simulink model "quadplane_sim"  (R2023a)
settings: Solver=FixedStepAuto  StartTime=0.0  StopTime=5  FixedStep=0.00001  RelTol=1e-6
values from neighbouring files (symbols this model uses):
  framePeriod_s = 1/frameRate_hz    (= 0.02)    [setup.m]
undefined symbols (not defined in the file or in its folder): Aircraft, datetime, datevec, Earth, Env, Fmu, InitCond, Telem, WGS84
libraries: simulink x9, aerolibconvert2 x5, aerolibasang x3, aerolibtransform2 x2, aerolibatmos2 x1, aerolibgravity2 x1, sharedtransform x1, uavutilslib x1, aerolibadyn x1, shared6dof x1
(part 4 of 4)

== system quadplane_sim/Flight Management Unit/Control Laws/Variant Subsystem/FMU v2/Virtual to Non-Virtual Mapping4/Subsystem2 ==
  Non-Virtual : Inport  OutDataTypeStr=Bus: AnalogData
  Bus Creator : BusCreator  Inputs=1
  Bus Selector : BusSelector  OutputSignals=val
  Data Type Conversion : DataTypeConversion  OutDataTypeStr=double  SaturateOnIntegerOverflow=off  RndMeth=Floor
  Virtual : Outport
  wires:
  Non-Virtual/1 -> Bus Selector/1
  Bus Creator/1 -> Virtual/1
  Data Type Conversion/1 -> Bus Creator/1  "Values"
  Bus Selector/1 -> Data Type Conversion/1  "<val>"

== system quadplane_sim/Flight Management Unit/Control Laws/Variant Subsystem/FMU v2/Virtual to Non-Virtual Mapping4/Subsystem3 ==
  Non-Virtual : Inport  OutDataTypeStr=Bus: PwmCmd
  Bus Creator : BusCreator  Inputs=2
  Bus Selector : BusSelector  OutputSignals=cnt,cmd
  Data Type Conversion : DataTypeConversion  OutDataTypeStr=double  SaturateOnIntegerOverflow=off  RndMeth=Floor
  Data Type Conversion1 : DataTypeConversion  OutDataTypeStr=double  SaturateOnIntegerOverflow=off  RndMeth=Floor
  Virtual : Outport
  wires:
  Non-Virtual/1 -> Bus Selector/1
  Bus Selector/2 -> Data Type Conversion1/1  "<cmd>"
  Data Type Conversion1/1 -> Bus Creator/2  "Cmds"
  Data Type Conversion/1 -> Bus Creator/1  "Cnt"
  Bus Selector/1 -> Data Type Conversion/1  "<cnt>"
  Bus Creator/1 -> Virtual/1

== system quadplane_sim/Flight Management Unit/Control Laws/Variant Subsystem/FMU v2/Virtual to Non-Virtual Mapping4/Subsystem4 ==
  Non-Virtual : Inport  OutDataTypeStr=Bus: SbusCmd
  Bus Creator : BusCreator  Inputs=4
  Bus Selector : BusSelector  OutputSignals=ch17,ch18,cnt,cmd
  Data Type Conversion{,1..3} (4 alike) : DataTypeConversion  OutDataTypeStr=double  SaturateOnIntegerOverflow=off  RndMeth=Floor
  Virtual : Outport
  wires:
  Non-Virtual/1 -> Bus Selector/1
  Bus Creator/1 -> Virtual/1
  Bus Selector/1 -> Data Type Conversion/1  "<ch17>"
  Bus Selector/2 -> Data Type Conversion1/1  "<ch18>"
  Bus Selector/3 -> Data Type Conversion2/1  "<cnt>"
  Bus Selector/4 -> Data Type Conversion3/1  "<cmd>"
  Data Type Conversion2/1 -> Bus Creator/3  "Cnt"
  Data Type Conversion3/1 -> Bus Creator/4  "Cmds"
  Data Type Conversion1/1 -> Bus Creator/2  "Ch 18"
  Data Type Conversion/1 -> Bus Creator/1  "Ch 17"

== system quadplane_sim/Flight Management Unit/Control Laws/Variant Subsystem/FMU v2/Virtual to Non-Virtual Mapping5/Virtual to Non-Virtual Mapping1 ==
  Virtual : Inport
  Bus Creator : BusCreator  Inputs=6
  Bus Selector : BusSelector  OutputSignals=New Data,Lost Frame,Failsafe,Ch 17,Ch 18,Channel Data
  Data Type Conversion{,1..4} (5 alike) : DataTypeConversion  OutDataTypeStr=boolean  SaturateOnIntegerOverflow=off  RndMeth=Floor
  Data Type Conversion5 : DataTypeConversion  OutDataTypeStr=int16  SaturateOnIntegerOverflow=off  RndMeth=Floor
  Non-Virtual : Outport  OutDataTypeStr=Bus: InceptorData
  wires:
  Virtual/1 -> Bus Selector/1
  Bus Creator/1 -> Non-Virtual/1
  Bus Selector/1 -> Data Type Conversion/1  "<New Data>"
  Bus Selector/2 -> Data Type Conversion1/1  "<Lost Frame>"
  Bus Selector/3 -> Data Type Conversion2/1  "<Failsafe>"
  Bus Selector/4 -> Data Type Conversion3/1  "<Ch 17>"
  Bus Selector/5 -> Data Type Conversion4/1  "<Ch 18>"
  Bus Selector/6 -> Data Type Conversion5/1  "<Channel Data>"
  Data Type Conversion/1 -> Bus Creator/1  "new_data"
  Data Type Conversion1/1 -> Bus Creator/2  "lost_frame"
  Data Type Conversion2/1 -> Bus Creator/3  "failsafe"
  Data Type Conversion3/1 -> Bus Creator/4  "ch17"
  Data Type Conversion4/1 -> Bus Creator/5  "ch18"
  Data Type Conversion5/1 -> Bus Creator/6  "ch"

== system quadplane_sim/Flight Management Unit/Control Laws/Variant Subsystem/FMU v2/Virtual to Non-Virtual Mapping5/Virtual to Non-Virtual Mapping2 ==
  Virtual : Inport
  Bus Creator : BusCreator  Inputs=8
  Bus Selector : BusSelector  OutputSignals=New IMU Data,New Magnetometer Data,IMU Healthy,Magnetometer Healthy,Die Temperature [C],Accelerometer [m/s/s],Gyro [rad/s],Magnetometer [uT]
  Data Type Conversion{,1..3} (4 alike) : DataTypeConversion  OutDataTypeStr=boolean  SaturateOnIntegerOverflow=off  RndMeth=Floor
  Data Type Conversion{4..7} (4 alike) : DataTypeConversion  OutDataTypeStr=single  SaturateOnIntegerOverflow=off  RndMeth=Floor
  Non-Virtual : Outport  OutDataTypeStr=Bus: ImuData
  wires:
  Bus Creator/1 -> Non-Virtual/1
  Virtual/1 -> Bus Selector/1
  Bus Selector/1 -> Data Type Conversion/1  "<New IMU Data>"
  Data Type Conversion/1 -> Bus Creator/1  "new_imu_data"
  Bus Selector/2 -> Data Type Conversion1/1  "<New Magnetometer Data>"
  Data Type Conversion1/1 -> Bus Creator/2  "new_mag_data"
  Bus Selector/3 -> Data Type Conversion2/1  "<IMU Healthy>"
  Data Type Conversion2/1 -> Bus Creator/3  "imu_healthy"
  Bus Selector/4 -> Data Type Conversion3/1  "<Magnetometer Healthy>"
  Data Type Conversion3/1 -> Bus Creator/4  "mag_healthy"
  Bus Selector/5 -> Data Type Conversion4/1  "<Die Temperature [C]>"
  Data Type Conversion4/1 -> Bus Creator/5  "die_temp_c"
  Bus Selector/6 -> Data Type Conversion5/1  "<Accelerometer [m/s/s]>"
  Bus Selector/7 -> Data Type Conversion6/1  "<Gyro [rad/s]>"
  Bus Selector/8 -> Data Type Conversion7/1  "<Magnetometer [uT]>"
  Data Type Conversion5/1 -> Bus Creator/6  "accel_mps2"
  Data Type Conversion6/1 -> Bus Creator/7  "gyro_radps"
  Data Type Conversion7/1 -> Bus Creator/8  "mag_ut"

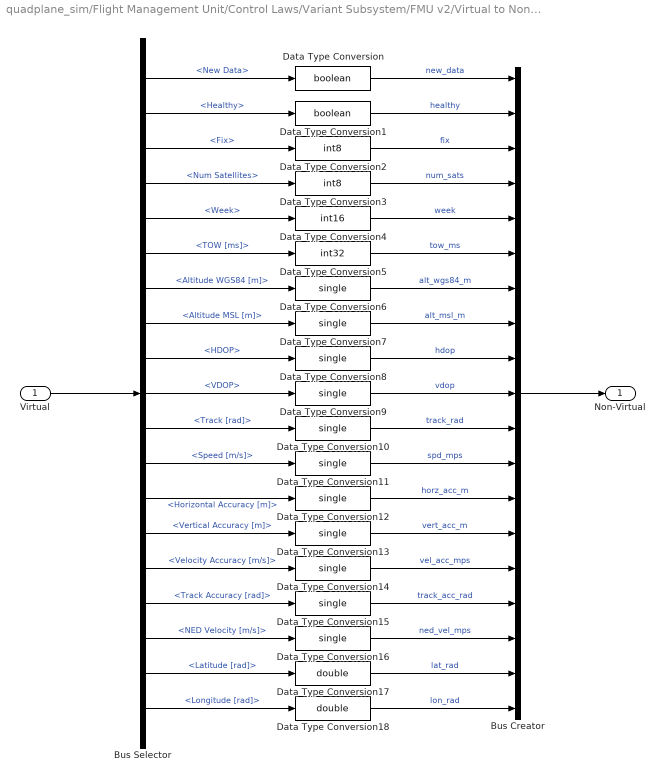
== system quadplane_sim/Flight Management Unit/Control Laws/Variant Subsystem/FMU v2/Virtual to Non-Virtual Mapping5/Virtual to Non-Virtual Mapping3 ==
  Virtual : Inport
  Bus Creator : BusCreator  Inputs=19
  Bus Selector : BusSelector  OutputSignals=New Data,Healthy,Fix,Num Satellites,Week,TOW [ms],Altitude WGS84 [m],Altitude MSL [m],HDOP,VDOP,Track [rad],Speed [m/s],Horizontal Accuracy [m],Vertical Accuracy [m],Velocity Accuracy [m/s],Track Accuracy [rad],NED Velocity [m/s],Latitude [rad],Longitude [rad]
  Data Type Conversion : DataTypeConversion  OutDataTypeStr=boolean  SaturateOnIntegerOverflow=off  RndMeth=Floor
  Data Type Conversion1 : DataTypeConversion  OutDataTypeStr=boolean  SaturateOnIntegerOverflow=off  RndMeth=Floor
  Data Type Conversion{6..16} (11 alike) : DataTypeConversion  OutDataTypeStr=single  SaturateOnIntegerOverflow=off  RndMeth=Floor
  Data Type Conversion17 : DataTypeConversion  OutDataTypeStr=double  SaturateOnIntegerOverflow=off  RndMeth=Floor
  Data Type Conversion18 : DataTypeConversion  OutDataTypeStr=double  SaturateOnIntegerOverflow=off  RndMeth=Floor
  Data Type Conversion2 : DataTypeConversion  OutDataTypeStr=int8  SaturateOnIntegerOverflow=off  RndMeth=Floor
  Data Type Conversion3 : DataTypeConversion  OutDataTypeStr=int8  SaturateOnIntegerOverflow=off  RndMeth=Floor
  Data Type Conversion4 : DataTypeConversion  OutDataTypeStr=int16  SaturateOnIntegerOverflow=off  RndMeth=Floor
  Data Type Conversion5 : DataTypeConversion  OutDataTypeStr=int32  SaturateOnIntegerOverflow=off  RndMeth=Floor
  Non-Virtual : Outport  OutDataTypeStr=Bus: GnssData
  wires:
  Virtual/1 -> Bus Selector/1
  Bus Creator/1 -> Non-Virtual/1
  Bus Selector/1 -> Data Type Conversion/1  "<New Data>"
  Data Type Conversion/1 -> Bus Creator/1  "new_data"
  Bus Selector/2 -> Data Type Conversion1/1  "<Healthy>"
  Data Type Conversion1/1 -> Bus Creator/2  "healthy"
  Bus Selector/3 -> Data Type Conversion2/1  "<Fix>"
  Data Type Conversion2/1 -> Bus Creator/3  "fix"
  Bus Selector/4 -> Data Type Conversion3/1  "<Num Satellites>"
  Data Type Conversion3/1 -> Bus Creator/4  "num_sats"
  Bus Selector/5 -> Data Type Conversion4/1  "<Week>"
  Data Type Conversion4/1 -> Bus Creator/5  "week"
  Bus Selector/6 -> Data Type Conversion5/1  "<TOW [ms]>"
  Data Type Conversion5/1 -> Bus Creator/6  "tow_ms"
  Bus Selector/7 -> Data Type Conversion6/1  "<Altitude WGS84 [m]>"
  Bus Selector/8 -> Data Type Conversion7/1  "<Altitude MSL [m]>"
  Data Type Conversion6/1 -> Bus Creator/7  "alt_wgs84_m"
  Data Type Conversion7/1 -> Bus Creator/8  "alt_msl_m"
  Bus Selector/9 -> Data Type Conversion8/1  "<HDOP>"
  Bus Selector/10 -> Data Type Conversion9/1  "<VDOP>"
  Data Type Conversion8/1 -> Bus Creator/9  "hdop"
  Data Type Conversion9/1 -> Bus Creator/10  "vdop"
  Bus Selector/11 -> Data Type Conversion10/1  "<Track [rad]>"
  Bus Selector/12 -> Data Type Conversion11/1  "<Speed [m/s]>"
  Data Type Conversion10/1 -> Bus Creator/11  "track_rad"
  Data Type Conversion11/1 -> Bus Creator/12  "spd_mps"
  Bus Selector/13 -> Data Type Conversion12/1  "<Horizontal Accuracy [m]>"
  Bus Selector/14 -> Data Type Conversion13/1  "<Vertical Accuracy [m]>"
  Bus Selector/15 -> Data Type Conversion14/1  "<Velocity Accuracy [m/s]>"
  Bus Selector/16 -> Data Type Conversion15/1  "<Track Accuracy [rad]>"
  Bus Selector/17 -> Data Type Conversion16/1  "<NED Velocity [m/s]>"
  Bus Selector/18 -> Data Type Conversion17/1  "<Latitude [rad]>"
  Bus Selector/19 -> Data Type Conversion18/1  "<Longitude [rad]>"
  Data Type Conversion18/1 -> Bus Creator/19  "lon_rad"
  Data Type Conversion17/1 -> Bus Creator/18  "lat_rad"
  Data Type Conversion16/1 -> Bus Creator/17  "ned_vel_mps"
  Data Type Conversion15/1 -> Bus Creator/16  "track_acc_rad"
  Data Type Conversion14/1 -> Bus Creator/15  "vel_acc_mps"
  Data Type Conversion13/1 -> Bus Creator/14  "vert_acc_m"
  Data Type Conversion12/1 -> Bus Creator/13  "horz_acc_m"

== system quadplane_sim/Flight Management Unit/Control Laws/Variant Subsystem/FMU v2/Virtual to Non-Virtual Mapping5/Virtual to Non-Virtual Mapping4 ==
  Virtual : Inport
  Bus Creator : BusCreator  Inputs=4
  Bus Selector : BusSelector  OutputSignals=New Data,Healthy,Pressure [Pa],Die Temperature [C]
  Data Type Conversion : DataTypeConversion  OutDataTypeStr=boolean  SaturateOnIntegerOverflow=off  RndMeth=Floor
  Data Type Conversion1 : DataTypeConversion  OutDataTypeStr=boolean  SaturateOnIntegerOverflow=off  RndMeth=Floor
  Data Type Conversion2 : DataTypeConversion  OutDataTypeStr=single  SaturateOnIntegerOverflow=off  RndMeth=Floor
  Data Type Conversion3 : DataTypeConversion  OutDataTypeStr=single  SaturateOnIntegerOverflow=off  RndMeth=Floor
  Non-Virtual : Outport  OutDataTypeStr=Bus: PresData
  wires:
  Bus Creator/1 -> Non-Virtual/1
  Virtual/1 -> Bus Selector/1
  Bus Selector/1 -> Data Type Conversion/1  "<New Data>"
  Data Type Conversion/1 -> Bus Creator/1  "new_data"
  Bus Selector/2 -> Data Type Conversion1/1  "<Healthy>"
  Data Type Conversion1/1 -> Bus Creator/2  "healthy"
  Bus Selector/3 -> Data Type Conversion2/1  "<Pressure [Pa]>"
  Data Type Conversion2/1 -> Bus Creator/3  "pres_pa"
  Bus Selector/4 -> Data Type Conversion3/1  "<Die Temperature [C]>"
  Data Type Conversion3/1 -> Bus Creator/4  "die_temp_c"

== system quadplane_sim/Flight Management Unit/Control Laws/Variant Subsystem/FMU v2/Virtual to Non-Virtual Mapping5/Virtual to Non-Virtual Mapping5 ==
  Virtual : Inport
  Bus Creator : BusCreator  Inputs=4
  Bus Selector : BusSelector  OutputSignals=New Data,Healthy,Pressure [Pa],Die Temperature [C]
  Data Type Conversion : DataTypeConversion  OutDataTypeStr=boolean  SaturateOnIntegerOverflow=off  RndMeth=Floor
  Data Type Conversion1 : DataTypeConversion  OutDataTypeStr=boolean  SaturateOnIntegerOverflow=off  RndMeth=Floor
  Data Type Conversion2 : DataTypeConversion  OutDataTypeStr=single  SaturateOnIntegerOverflow=off  RndMeth=Floor
  Data Type Conversion3 : DataTypeConversion  OutDataTypeStr=single  SaturateOnIntegerOverflow=off  RndMeth=Floor
  Non-Virtual : Outport  OutDataTypeStr=Bus: PresData
  wires:
  Data Type Conversion3/1 -> Bus Creator/4  "die_temp_c"
  Bus Selector/4 -> Data Type Conversion3/1  "<Die Temperature [C]>"
  Data Type Conversion2/1 -> Bus Creator/3  "pres_pa"
  Bus Selector/3 -> Data Type Conversion2/1  "<Pressure [Pa]>"
  Data Type Conversion1/1 -> Bus Creator/2  "healthy"
  Bus Selector/2 -> Data Type Conversion1/1  "<Healthy>"
  Data Type Conversion/1 -> Bus Creator/1  "new_data"
  Bus Selector/1 -> Data Type Conversion/1  "<New Data>"
  Virtual/1 -> Bus Selector/1
  Bus Creator/1 -> Non-Virtual/1

== system quadplane_sim/Flight Management Unit/Control Laws/Variant Subsystem/FMU v2/Virtual to Non-Virtual Mapping5/Virtual to Non-Virtual Mapping6 ==
  Virtual : Inport
  Bus Creator : BusCreator  Inputs=1
  Bus Selector : BusSelector  OutputSignals=Voltages
  Data Type Conversion2 : DataTypeConversion  OutDataTypeStr=single  SaturateOnIntegerOverflow=off  RndMeth=Floor
  Non-Virtual : Outport  OutDataTypeStr=Bus: AdcData
  wires:
  Bus Creator/1 -> Non-Virtual/1
  Virtual/1 -> Bus Selector/1
  Data Type Conversion2/1 -> Bus Creator/1  "volt"
  Bus Selector/1 -> Data Type Conversion2/1  "<Voltages>"

== system quadplane_sim/Flight Management Unit/Control Laws/Variant Subsystem/FMU v2/Virtual to Non-Virtual Mapping5/Virtual to Non-Virtual Mapping7 ==
  Virtual : Inport
  Bus Creator : BusCreator  Inputs=2
  Bus Selector : BusSelector  OutputSignals=Voltage [V],Current [V]
  Data Type Conversion1 : DataTypeConversion  OutDataTypeStr=single  SaturateOnIntegerOverflow=off  RndMeth=Floor
  Data Type Conversion2 : DataTypeConversion  OutDataTypeStr=single  SaturateOnIntegerOverflow=off  RndMeth=Floor
  Non-Virtual : Outport  OutDataTypeStr=Bus: PowerModuleData
  wires:
  Virtual/1 -> Bus Selector/1
  Bus Creator/1 -> Non-Virtual/1
  Bus Selector/1 -> Data Type Conversion1/1  "<Voltage [V]>"
  Data Type Conversion1/1 -> Bus Creator/1  "voltage_v"
  Bus Selector/2 -> Data Type Conversion2/1  "<Current [V]>"
  Data Type Conversion2/1 -> Bus Creator/2  "current_v"

== system quadplane_sim/Flight Management Unit/Control Laws/Variant Subsystem/FMU v2 Beta/Virtual to Non-Virtual Mapping1/Virtual to Non-Virtual Mapping1 ==
  Virtual : Inport
  Bus Creator : BusCreator  Inputs=10
  Bus Selector : BusSelector  OutputSignals=New Data,Lost Frame,Failsafe,Throttle Enable,Mode 0,Mode 1,Throttle,Pitch,Pitch,Yaw
  Data Type Conversion{,1..3} (4 alike) : DataTypeConversion  OutDataTypeStr=boolean  SaturateOnIntegerOverflow=off  RndMeth=Floor
  Data Type Conversion4 : DataTypeConversion  OutDataTypeStr=int8  SaturateOnIntegerOverflow=off  RndMeth=Floor
  Data Type Conversion5 : DataTypeConversion  OutDataTypeStr=int8  SaturateOnIntegerOverflow=off  RndMeth=Floor
  Data Type Conversion{6..9} (4 alike) : DataTypeConversion  OutDataTypeStr=single  SaturateOnIntegerOverflow=off  RndMeth=Floor
  Non-Virtual : Outport  OutDataTypeStr=Bus: InceptorData
  wires:
  Virtual/1 -> Bus Selector/1
  Bus Creator/1 -> Non-Virtual/1
  Bus Selector/1 -> Data Type Conversion/1  "<New Data>"
  Data Type Conversion/1 -> Bus Creator/1  "new_data"
  Bus Selector/2 -> Data Type Conversion1/1  "<Lost Frame>"
  Bus Selector/3 -> Data Type Conversion2/1  "<Failsafe>"
  Bus Selector/4 -> Data Type Conversion3/1  "<Throttle Enable>"
  Bus Selector/5 -> Data Type Conversion4/1  "<Mode 0>"
  Bus Selector/6 -> Data Type Conversion5/1  "<Mode 1>"
  Bus Selector/7 -> Data Type Conversion6/1  "<Throttle>"
  Bus Selector/8 -> Data Type Conversion7/1  "<Pitch>"
  Bus Selector/9 -> Data Type Conversion8/1  "<Pitch>"
  Bus Selector/10 -> Data Type Conversion9/1  "<Yaw>"
  Data Type Conversion1/1 -> Bus Creator/2  "lost_frame"
  Data Type Conversion2/1 -> Bus Creator/3  "failsafe"
  Data Type Conversion3/1 -> Bus Creator/4  "throttle_en"
  Data Type Conversion4/1 -> Bus Creator/5  "mode0"
  Data Type Conversion5/1 -> Bus Creator/6  "mode1"
  Data Type Conversion6/1 -> Bus Creator/7  "throttle"
  Data Type Conversion7/1 -> Bus Creator/8  "pitch"
  Data Type Conversion8/1 -> Bus Creator/9  "roll"
  Data Type Conversion9/1 -> Bus Creator/10  "yaw"

== system quadplane_sim/Flight Management Unit/Control Laws/Variant Subsystem/FMU v2 Beta/Virtual to Non-Virtual Mapping1/Virtual to Non-Virtual Mapping2 ==
  Virtual : Inport
  Bus Creator : BusCreator  Inputs=8
  Bus Selector : BusSelector  OutputSignals=New IMU Data,New Magnetometer Data,IMU Healthy,Magnetometer Healthy,Die Temperature [C],Accelerometer [m/s/s],Gyro [rad/s],Magnetometer [uT]
  Data Type Conversion{,1..3} (4 alike) : DataTypeConversion  OutDataTypeStr=boolean  SaturateOnIntegerOverflow=off  RndMeth=Floor
  Data Type Conversion{4..7} (4 alike) : DataTypeConversion  OutDataTypeStr=single  SaturateOnIntegerOverflow=off  RndMeth=Floor
  Non-Virtual : Outport  OutDataTypeStr=Bus: ImuData
  wires:
  Bus Creator/1 -> Non-Virtual/1
  Virtual/1 -> Bus Selector/1
  Bus Selector/1 -> Data Type Conversion/1  "<New IMU Data>"
  Data Type Conversion/1 -> Bus Creator/1  "new_imu_data"
  Bus Selector/2 -> Data Type Conversion1/1  "<New Magnetometer Data>"
  Data Type Conversion1/1 -> Bus Creator/2  "new_mag_data"
  Bus Selector/3 -> Data Type Conversion2/1  "<IMU Healthy>"
  Data Type Conversion2/1 -> Bus Creator/3  "imu_healthy"
  Bus Selector/4 -> Data Type Conversion3/1  "<Magnetometer Healthy>"
  Data Type Conversion3/1 -> Bus Creator/4  "mag_healthy"
  Bus Selector/5 -> Data Type Conversion4/1  "<Die Temperature [C]>"
  Data Type Conversion4/1 -> Bus Creator/5  "die_temp_c"
  Bus Selector/6 -> Data Type Conversion5/1  "<Accelerometer [m/s/s]>"
  Bus Selector/7 -> Data Type Conversion6/1  "<Gyro [rad/s]>"
  Bus Selector/8 -> Data Type Conversion7/1  "<Magnetometer [uT]>"
  Data Type Conversion5/1 -> Bus Creator/6  "accel_mps2"
  Data Type Conversion6/1 -> Bus Creator/7  "gyro_radps"
  Data Type Conversion7/1 -> Bus Creator/8  "mag_ut"

== system quadplane_sim/Flight Management Unit/Control Laws/Variant Subsystem/FMU v2 Beta/Virtual to Non-Virtual Mapping1/Virtual to Non-Virtual Mapping3 ==
  Virtual : Inport
  Bus Creator : BusCreator  Inputs=19
  Bus Selector : BusSelector  OutputSignals=New Data,Healthy,Fix,Num Satellites,Week,TOW [ms],Altitude WGS84 [m],Altitude MSL [m],HDOP,VDOP,Track [rad],Speed [m/s],Horizontal Accuracy [m],Vertical Accuracy [m],Velocity Accuracy [m/s],Track Accuracy [rad],NED Velocity [m/s],Latitude [rad],Longitude [rad]
  Data Type Conversion : DataTypeConversion  OutDataTypeStr=boolean  SaturateOnIntegerOverflow=off  RndMeth=Floor
  Data Type Conversion1 : DataTypeConversion  OutDataTypeStr=boolean  SaturateOnIntegerOverflow=off  RndMeth=Floor
  Data Type Conversion{6..16} (11 alike) : DataTypeConversion  OutDataTypeStr=single  SaturateOnIntegerOverflow=off  RndMeth=Floor
  Data Type Conversion17 : DataTypeConversion  OutDataTypeStr=double  SaturateOnIntegerOverflow=off  RndMeth=Floor
  Data Type Conversion18 : DataTypeConversion  OutDataTypeStr=double  SaturateOnIntegerOverflow=off  RndMeth=Floor
  Data Type Conversion2 : DataTypeConversion  OutDataTypeStr=int8  SaturateOnIntegerOverflow=off  RndMeth=Floor
  Data Type Conversion3 : DataTypeConversion  OutDataTypeStr=int8  SaturateOnIntegerOverflow=off  RndMeth=Floor
  Data Type Conversion4 : DataTypeConversion  OutDataTypeStr=int16  SaturateOnIntegerOverflow=off  RndMeth=Floor
  Data Type Conversion5 : DataTypeConversion  OutDataTypeStr=int32  SaturateOnIntegerOverflow=off  RndMeth=Floor
  Non-Virtual : Outport  OutDataTypeStr=Bus: GnssData
  wires:
  Virtual/1 -> Bus Selector/1
  Bus Creator/1 -> Non-Virtual/1
  Bus Selector/1 -> Data Type Conversion/1  "<New Data>"
  Data Type Conversion/1 -> Bus Creator/1  "new_data"
  Bus Selector/2 -> Data Type Conversion1/1  "<Healthy>"
  Data Type Conversion1/1 -> Bus Creator/2  "healthy"
  Bus Selector/3 -> Data Type Conversion2/1  "<Fix>"
  Data Type Conversion2/1 -> Bus Creator/3  "fix"
  Bus Selector/4 -> Data Type Conversion3/1  "<Num Satellites>"
  Data Type Conversion3/1 -> Bus Creator/4  "num_sats"
  Bus Selector/5 -> Data Type Conversion4/1  "<Week>"
  Data Type Conversion4/1 -> Bus Creator/5  "week"
  Bus Selector/6 -> Data Type Conversion5/1  "<TOW [ms]>"
  Data Type Conversion5/1 -> Bus Creator/6  "tow_ms"
  Bus Selector/7 -> Data Type Conversion6/1  "<Altitude WGS84 [m]>"
  Bus Selector/8 -> Data Type Conversion7/1  "<Altitude MSL [m]>"
  Data Type Conversion6/1 -> Bus Creator/7  "alt_wgs84_m"
  Data Type Conversion7/1 -> Bus Creator/8  "alt_msl_m"
  Bus Selector/9 -> Data Type Conversion8/1  "<HDOP>"
  Bus Selector/10 -> Data Type Conversion9/1  "<VDOP>"
  Data Type Conversion8/1 -> Bus Creator/9  "hdop"
  Data Type Conversion9/1 -> Bus Creator/10  "vdop"
  Bus Selector/11 -> Data Type Conversion10/1  "<Track [rad]>"
  Bus Selector/12 -> Data Type Conversion11/1  "<Speed [m/s]>"
  Data Type Conversion10/1 -> Bus Creator/11  "track_rad"
  Data Type Conversion11/1 -> Bus Creator/12  "spd_mps"
  Bus Selector/13 -> Data Type Conversion12/1  "<Horizontal Accuracy [m]>"
  Bus Selector/14 -> Data Type Conversion13/1  "<Vertical Accuracy [m]>"
  Bus Selector/15 -> Data Type Conversion14/1  "<Velocity Accuracy [m/s]>"
  Bus Selector/16 -> Data Type Conversion15/1  "<Track Accuracy [rad]>"
  Bus Selector/17 -> Data Type Conversion16/1  "<NED Velocity [m/s]>"
  Bus Selector/18 -> Data Type Conversion17/1  "<Latitude [rad]>"
  Bus Selector/19 -> Data Type Conversion18/1  "<Longitude [rad]>"
  Data Type Conversion18/1 -> Bus Creator/19  "lon_rad"
  Data Type Conversion17/1 -> Bus Creator/18  "lat_rad"
  Data Type Conversion16/1 -> Bus Creator/17  "ned_vel_mps"
  Data Type Conversion15/1 -> Bus Creator/16  "track_acc_rad"
  Data Type Conversion14/1 -> Bus Creator/15  "vel_acc_mps"
  Data Type Conversion13/1 -> Bus Creator/14  "vert_acc_m"
  Data Type Conversion12/1 -> Bus Creator/13  "horz_acc_m"

== system quadplane_sim/Flight Management Unit/Control Laws/Variant Subsystem/FMU v2 Beta/Virtual to Non-Virtual Mapping1/Virtual to Non-Virtual Mapping4 ==
  Virtual : Inport
  Bus Creator : BusCreator  Inputs=4
  Bus Selector : BusSelector  OutputSignals=New Data,Healthy,Pressure [Pa],Die Temperature [C]
  Data Type Conversion : DataTypeConversion  OutDataTypeStr=boolean  SaturateOnIntegerOverflow=off  RndMeth=Floor
  Data Type Conversion1 : DataTypeConversion  OutDataTypeStr=boolean  SaturateOnIntegerOverflow=off  RndMeth=Floor
  Data Type Conversion2 : DataTypeConversion  OutDataTypeStr=single  SaturateOnIntegerOverflow=off  RndMeth=Floor
  Data Type Conversion3 : DataTypeConversion  OutDataTypeStr=single  SaturateOnIntegerOverflow=off  RndMeth=Floor
  Non-Virtual : Outport  OutDataTypeStr=Bus: PresData
  wires:
  Bus Creator/1 -> Non-Virtual/1
  Virtual/1 -> Bus Selector/1
  Bus Selector/1 -> Data Type Conversion/1  "<New Data>"
  Data Type Conversion/1 -> Bus Creator/1  "new_data"
  Bus Selector/2 -> Data Type Conversion1/1  "<Healthy>"
  Data Type Conversion1/1 -> Bus Creator/2  "healthy"
  Bus Selector/3 -> Data Type Conversion2/1  "<Pressure [Pa]>"
  Data Type Conversion2/1 -> Bus Creator/3  "pres_pa"
  Bus Selector/4 -> Data Type Conversion3/1  "<Die Temperature [C]>"
  Data Type Conversion3/1 -> Bus Creator/4  "die_temp_c"

== system quadplane_sim/Flight Management Unit/Control Laws/Variant Subsystem/FMU v2 Beta/Virtual to Non-Virtual Mapping1/Virtual to Non-Virtual Mapping5 ==
  Virtual : Inport
  Bus Creator : BusCreator  Inputs=4
  Bus Selector : BusSelector  OutputSignals=New Data,Healthy,Pressure [Pa],Die Temperature [C]
  Data Type Conversion : DataTypeConversion  OutDataTypeStr=boolean  SaturateOnIntegerOverflow=off  RndMeth=Floor
  Data Type Conversion1 : DataTypeConversion  OutDataTypeStr=boolean  SaturateOnIntegerOverflow=off  RndMeth=Floor
  Data Type Conversion2 : DataTypeConversion  OutDataTypeStr=single  SaturateOnIntegerOverflow=off  RndMeth=Floor
  Data Type Conversion3 : DataTypeConversion  OutDataTypeStr=single  SaturateOnIntegerOverflow=off  RndMeth=Floor
  Non-Virtual : Outport  OutDataTypeStr=Bus: PresData
  wires:
  Data Type Conversion3/1 -> Bus Creator/4  "die_temp_c"
  Bus Selector/4 -> Data Type Conversion3/1  "<Die Temperature [C]>"
  Data Type Conversion2/1 -> Bus Creator/3  "pres_pa"
  Bus Selector/3 -> Data Type Conversion2/1  "<Pressure [Pa]>"
  Data Type Conversion1/1 -> Bus Creator/2  "healthy"
  Bus Selector/2 -> Data Type Conversion1/1  "<Healthy>"
  Data Type Conversion/1 -> Bus Creator/1  "new_data"
  Bus Selector/1 -> Data Type Conversion/1  "<New Data>"
  Virtual/1 -> Bus Selector/1
  Bus Creator/1 -> Non-Virtual/1

== system quadplane_sim/Flight Management Unit/Control Laws/Variant Subsystem/FMU v2 Beta/Virtual to Non-Virtual Mapping1/Virtual to Non-Virtual Mapping6 ==
  Virtual : Inport
  Bus Creator : BusCreator  Inputs=2
  Bus Selector : BusSelector  OutputSignals=Voltages,Values
  Data Type Conversion2 : DataTypeConversion  OutDataTypeStr=single  SaturateOnIntegerOverflow=off  RndMeth=Floor
  Data Type Conversion3 : DataTypeConversion  OutDataTypeStr=single  SaturateOnIntegerOverflow=off  RndMeth=Floor
  Non-Virtual : Outport  OutDataTypeStr=Bus: AnalogData
  wires:
  Bus Creator/1 -> Non-Virtual/1
  Virtual/1 -> Bus Selector/1
  Data Type Conversion2/1 -> Bus Creator/1  "volt"
  Bus Selector/1 -> Data Type Conversion2/1  "<Voltages>"
  Bus Selector/2 -> Data Type Conversion3/1  "<Values>"
  Data Type Conversion3/1 -> Bus Creator/2  "val"

== matlab function quadplane_sim/Vehicle/Forces and Moments/Propulsive/Forward Propulsion/Gyroscopic moment ==
  data: body_rotation input; motor_dir input; prop_rotation input; J input; Mxyz_gyro output; forward_index input
function Mxyz_gyro = gyro_moment(body_rotation, motor_dir, prop_rotation, J, forward_index)
% Calculates the gyroscopic moment from the propeller. 
% This is not included in the multirotor sim because this effect is ~
% cancelled by rotors spinning in opposite direction. 
% See Stevens Aircraft Control and Simulation Textbook

% Including terms J*w_prop, motor spin direction. Assuming the propeller is
% spinning about the x axis. 
term1 = - J * prop_rotation * motor_dir(forward_index);

% term for gyroscopic moment (Mxyz on body frame)
Mxyz_gyro = cross(body_rotation, [term1, 0, 0]);

== matlab function quadplane_sim/Vehicle/Forces and Moments/Aerodynamic/Forward Flight/Calculate Aerodynamic Coefficients ==
  data: alpha input; aero_coefs output; pqr input; deflections input; beta input
function aero_coefs = calculate_coefficients(alpha, pqr, deflections, beta)

% deflections are [left_ail, right_ail, elev, rudder]

% CL, CD, Cm are functions of (alpha, beta, elevator_def)
% CY, Cl, Cn are functions of (beta, p, q, r, aileron_def, rudder_def)
% all equations have a intercept term (example: CLo) and a linear slope
% term for each parameter (example: CL_alpha * alpha)

% Lift
CL = Aircraft.Aero.CL.zero + Aircraft.Aero.CL.alpha * alpha + ...
    Aircraft.Aero.CL.q * pqr(2) + Aircraft.Aero.CL.elevator_def * deflections(3);

% Drag
CD = Aircraft.Aero.CD.zero + Aircraft.Aero.CD.alpha * alpha + ...
    Aircraft.Aero.CD.q * pqr(2) + Aircraft.Aero.CD.elevator_def * deflections(3);

% Side Force
% assume aileron deflection to be symmetrical and in opposite direction
CY = Aircraft.Aero.CY.zero + Aircraft.Aero.CY.beta * beta + ...
    Aircraft.Aero.CY.p * pqr(1) + Aircraft.Aero.CY.q * pqr(2) + ...
    Aircraft.Aero.CY.r * pqr(3) + Aircraft.Aero.CY.aileron_def * ...
    deflections(1) + Aircraft.Aero.CY.rudder_def * deflections(4);

% Rolling moment 
Cl = Aircraft.Aero.Cl.zero + Aircraft.Aero.Cl.beta * beta + ...
    Aircraft.Aero.Cl.p * pqr(1) + Aircraft.Aero.Cl.q * pqr(2) + ...
    Aircraft.Aero.Cl.r * pqr(3) + Aircraft.Aero.Cl.aileron_def * ...
    deflections(1) + Aircraft.Aero.Cl.rudder_def * deflections(4);

% Pitching moment 
Cm = Aircraft.Aero.Cm.zero + Aircraft.Aero.Cm.alpha * alpha + ...
    Aircraft.Aero.Cm.q * pqr(2) + Aircraft.Aero.Cm.elevator_def * deflections(3);

% Yawing moment 
Cn = Aircraft.Aero.Cn.zero + Aircraft.Aero.Cn.beta * beta + ...
    Aircraft.Aero.Cn.p * pqr(1) + Aircraft.Aero.Cn.q * pqr(2) + ...
    Aircraft.Aero.Cn.r * pqr(3) + Aircraft.Aero.Cn.aileron_def * ...
    deflections(1) + Aircraft.Aero.Cn.rudder_def * deflections(4);

aero_coefs = [CL, CD, CY, Cl, Cm, Cn];

== matlab function quadplane_sim/Flight Management Unit/Sensor Models/GNSS/Triggered Subsystem/MATLAB Function ==
  data: year input; month input; mday input; hour input; minute input; second input; gnss_week output; sim_clock input; gnss_tow output
function [gnss_week, gnss_tow] = GnssWeekAndTime(year, month, mday, hour, minute, second, sim_clock)

JAN61980 = 44244;
JAN11901 = 15385;
SEC_PER_DAY = 86400.0;

month_day = [
    0, 31, 59, 90, 120, 151, 181, 212, 243, 273, 304, 334;
    0, 31, 60, 91, 121, 152, 182, 213, 244, 274, 305, 335
];

second = second + sim_clock;
leap = (mod(year,4) == 0);
yday = month_day(leap + 1, month) + mday;
mjd = ((year - 1901) / 4) * 1461 + mod((year - 1901), 4) * 365 + yday - 1 + JAN11901;
fmjd = ((second / 60.0 + minute) / 60.0 + hour) / 24.0;
gnss_week = floor((mjd - JAN61980) / 7);
gnss_tow = ((mjd - JAN61980) - gnss_week * 7 + fmjd) * SEC_PER_DAY;

== matlab function quadplane_sim/Flight Management Unit/Sensor Models/GNSS/Triggered Subsystem/MATLAB Function1 ==
  data: ang input; ret output
function ret  = constrain360(ang)
%Constrain360 Converts a +/-180 value to a 0 - 360 value
ret = fmod(ang, 360);
if ret < 0
    ret = ret + 360;
end

end

== matlab function quadplane_sim/Vehicle/Forces and Moments/Propulsive/Forward Propulsion/Motor Dynamics ==
  data: total_voltage input; motor_kv input; motor_io input; motor_r input; motor_cmd input; torque_Nm output; rotational_rate input
function torque_Nm = motor(total_voltage, motor_kv, motor_io, motor_r, motor_cmd, rotational_rate)
% Calculates the torque by the motor based on rotational rate and throttle
% cmd

% Effective voltage is essentially throttle % of total voltage supplied to
% the motor. This is used as input to the motor.
% https://electronics.stackexchange.com/questions/354155/what-does-changing
% -the-throttle-to-a-bldc-esc-actually-do
effective_voltage = motor_cmd * total_voltage;
kv = motor_kv * 2 * pi / 60;

% Look at simulations/references/motor_prop.pdf
inner_term = (effective_voltage - rotational_rate / kv) / motor_r;
torque_Nm = (inner_term - motor_io) / kv;

end

== matlab function quadplane_sim/Vehicle/Forces and Moments/Propulsive/Forward Propulsion/Propeller Dynamics ==
  data: airspeed input; moment_Nm output; density input; prop_rotational_rate input; thrust_N output; diameter_in input; ct_fit input; cp_fit input
function [moment_Nm, thrust_N]  = propeller(airspeed, density, prop_rotational_rate, diameter_in, ct_fit, cp_fit)
% Calculating thrust and torque from the motor

% manually converting in to m. (convlength is not supported for some reason.)
prop_radius = diameter_in * 0.0254 / 2;

% Advance ratio of propeller
lambda = airspeed / (prop_rotational_rate * prop_radius);

% thrust coefficient
ct = polyval(ct_fit, lambda);
% power coefficient
cp = polyval(cp_fit, lambda);

thrust_N = 0.5 * density * prop_rotational_rate^2 * pi * prop_radius^4 * ct;
moment_Nm = 0.5 * density * prop_rotational_rate^2 * pi * prop_radius^5 * cp;

end

== matlab function quadplane_sim/Vehicle/Forces and Moments/Propulsive/Hover Propulsion/Motor Model ==
  data: motor_thrust output; poly_thrust input; poly_torque input; dir input; align input; forward_bool input; Fxyz_motor output; Motor_cmd input; Mxyz_motor output
function [motor_thrust,Fxyz_motor,Mxyz_motor] = motor_model(poly_thrust, poly_torque, dir, align, forward_bool, Motor_cmd)

% Motor commands (only for hover)
% Thrust and torque polynomial fits based on input throttle (0-1)
% 1-by-5 thrust and torques

motor_thrust  = polyval(poly_thrust,Motor_cmd);
motor_torque  = polyval(poly_torque,Motor_cmd);

% neglecting the forward motor's contribution
motor_thrust = (1 - forward_bool)' .* motor_thrust;
motor_torque = (1 - forward_bool)' .* motor_torque;

% matrix multiply with the hover motors alignment to get total thrust and
% moment
% 1-by-3 Fxyz
Fxyz_motor = motor_thrust * align;

% adding all torques based on motor spinning direction
% Dot product with negative of hover motor directions to get each motor's
% torque.
% Cross product with the motor alignment to get the torque on boxy xyz
% Returns a 1-by-3 Mxyz vector
Mxyz_motor = (motor_torque .* -dir') * abs(align);


end

== matlab function quadplane_sim/Vehicle/Forces and Moments/Propulsive/Hover Propulsion/Moment From thrust arm ==
  data: cg_pos input; motor_pos input; nMotor input; align input; motor_thrust input; Mxyz_from_thrust output
function Mxyz_from_thrust = thrust_to_moment(cg_pos,motor_pos, nMotor, align, motor_thrust)
% Calculate the moment from the motors about cg.
% Returns 1-by-3 vector Mxyz

% 5-by-3 thrust from all motors in body xyz
all_motors_thrust = motor_thrust' .* align;

% calculating the moment arm for each motor
moment_arm = motor_pos - cg_pos';

moments_from_each_motor = zeros(5, 3);
Mxyz_from_thrust = zeros(1, 3);

for i = 1:nMotor

    % [Mx My Mz] for each motor
    moments_from_each_motor(i, :) = cross(moment_arm(i, :), all_motors_thrust(i, :));
    
    % [Mx My Mz] for all motors
    Mxyz_from_thrust = Mxyz_from_thrust + moments_from_each_motor(i, :);
end

end

== matlab function quadplane_sim/Vehicle/Forces and Moments/Propulsive/Forward Propulsion/Body Forces and Moments ==
  data: forward_index input; Fxyz_thrust output; motor_align input; cg_pos input; motor_pos input; motor_thrust input; Mxyz_thrust output; h_dot input; motor_dir input
function [Fxyz_thrust, Mxyz_thrust] = body_calcs(forward_index, motor_align, cg_pos,motor_pos,motor_thrust, h_dot, motor_dir)
% Calculate the moment from the motors about cg.
% Returns 1-by-3 vector Mxyz

% applying the direction of thrust based on motor alignment
Fxyz_thrust = motor_thrust * motor_align(forward_index, :);

% rate of change of angular momentum until equilibrium is reached between
% propeller and motor.
Mxyz_prop_motor = - h_dot * motor_dir(forward_index) * motor_align(forward_index, :);

% Moment about cg if the thrust has offset from cg. 
moment_arm = motor_pos(forward_index, :) - cg_pos';
Mxyz_thrust = Mxyz_prop_motor + cross(moment_arm, Fxyz_thrust);

end
